simulink model "pendulo"  (R2014a)
settings: Solver=ode3  StartTime=0.0  StopTime=ts  FixedStep=tm  RelTol=1e-3
values from neighbouring files (symbols this model uses):
  AA = [0 1;-(g/ele)*cos(x1t)-(k*a^2/(m*ele^2)*(cos(x1t)^2-sin(x1t)^2)) -b/(m*ele^2)]    [ejemnlin1.m]
  BB = [0; 1/(m*ele^2)]    [ejemnlin1.m]
  CC = [1 0;0 1 ]    [ejemnlin1.m]
  DD = [0;0]    [ejemnlin1.m]
  te = 0*pi/180    (= 0)    [ejemnlin1.m]
  ut = (g*m*ele)*sin(x1t) + (k*a^2)*sin(x1t)*cos(x1t) + b*x2t    [ejemnlin1.m]
  w = 10    [ejemnlin1.m]
  x10 = 20*pi/180    (= 0.349065850399)    [ejemnlin1.m]
  x1t = 20*pi/180    (= 0.349065850399)    [ejemnlin1.m]
  x20 = 0    [ejemnlin1.m]
  x2t = 0    [ejemnlin1.m]
  XL0 = [x10;x20] - [x1t;x2t]    [ejemnlin1.m]
  xm = 15    [ejemnlin1.m]
settings Model: Creator=mau  LastModifiedBy=mau

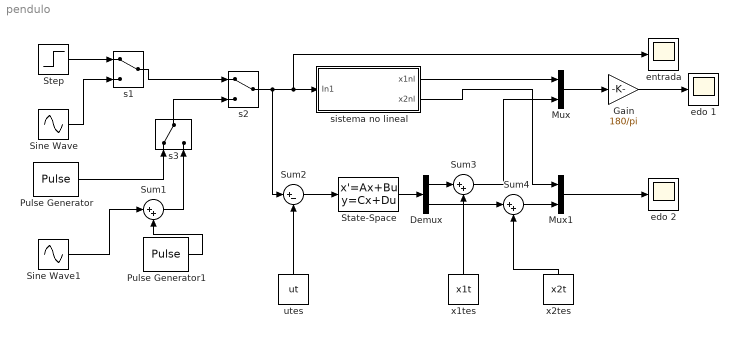
== system pendulo ==
  Demux : Demux  Outputs=2
  Gain : Gain  Gain=180/pi
  Mux : Mux  Inputs=2
  Mux1 : Mux  Inputs=2
  Pulse Generator : DiscretePulseGenerator  PulseType=Time based  Amplitude=xm  Period=50  PulseWidth=50
  Pulse Generator1 : DiscretePulseGenerator  PulseType=Time based  Amplitude=1.5  Period=50  PulseWidth=50
  Sine Wave : Sin  Amplitude=xm  Frequency=w  Phase=te  SampleTime=0
  Sine Wave1 : Sin  Amplitude=xm  Frequency=w  Phase=te  SampleTime=0
  State-Space : StateSpace  A=AA  B=BB  C=CC  D=DD  X0=XL0
  Step : Step  Time=0  After=xm  SampleTime=0
  Sum1 : Sum  Inputs=|++
  Sum2 : Sum  Inputs=|+-
  Sum3 : Sum  Inputs=|++
  Sum4 : Sum  Inputs=|++
  edo 1 : Scope
      settings: YMin=-10  YMax=15
  edo 2 : Scope
  entrada : Scope
      settings: YMin=-20  YMax=17.5  SaveName=ScopeData2
  s1 : ManualSwitch
  s2 : ManualSwitch
  s3 : ManualSwitch
  sistema no lineal : Subsystem  TreatAsAtomicUnit=on
  utes : Constant  Value=ut
  x1tes : Constant  Value=x1t
  x2tes : Constant  Value=x2t
  wires:
  Step/1 -> s1/1
  Sine Wave/1 -> s1/2
  s1/1 -> s2/1
  Sine Wave1/1 -> Sum1/1
  Pulse Generator1/1 -> Sum1/2
  Pulse Generator/1 -> s3/1
  s3/1 -> s2/2
  Sum1/1 -> s3/2
  s2/1 -> Sum2/1, entrada/1, sistema no lineal/1(In1)
  sistema no lineal/1(x1nl) -> Mux/1
  Mux/1 -> Gain/1
  State-Space/1 -> Demux/1
  sistema no lineal/2(x2nl) -> Mux1/1
  Mux1/1 -> edo 2/1
  utes/1 -> Sum2/2
  Sum2/1 -> State-Space/1
  Demux/1 -> Sum3/1
  Demux/2 -> Sum4/1
  Sum4/1 -> Mux1/2
  Sum3/1 -> Mux/2
  x1tes/1 -> Sum3/2
  x2tes/1 -> Sum4/2
  Gain/1 -> edo 1/1

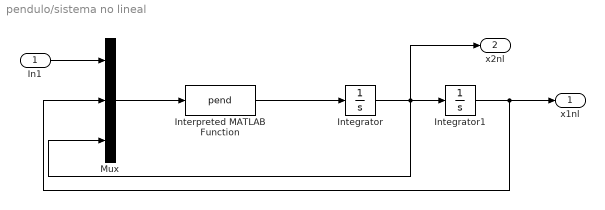
== system pendulo/sistema no lineal ==
  In1 : Inport
  Integrator : Integrator  InitialCondition=x20
  Integrator1 : Integrator  InitialCondition=x10
  Interpreted MATLAB Function : MATLABFcn  MATLABFcn=pend  OutputDimensions=1
  Mux : Mux  Inputs=3
  x1nl : Outport
  x2nl : Outport  Port=2
  wires:
  In1/1 -> Mux/1
  Integrator/1 -> Mux/3, x2nl/1, Integrator1/1
  Integrator1/1 -> Mux/2, x1nl/1
  Interpreted MATLAB Function/1 -> Integrator/1
  Mux/1 -> Interpreted MATLAB Function/1
